simulink model "KV_Function_Valve"  (R2013b)
settings: Solver=ode45  StartTime=0.0  StopTime=10.0  RelTol=1e-3
libraries: simulink x1
settings Model: Creator=drhf  LastModifiedBy=drhf
settings OptimizationCC: InlineParams=on

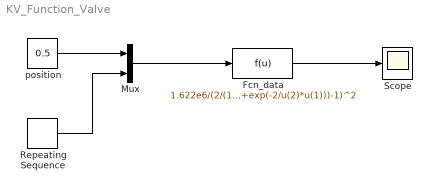
== system KV_Function_Valve ==
  Fcn_data : Fcn  Expr=1.622e6/(2/(1+exp(-2/u(2)*u(1)))-1)^2
  Mux : Mux  Inputs=2
  Repeating Sequence : simulink/Sources/Repeating Sequence  rep_seq_t=[0 10]  rep_seq_y=[0.5 10]
  Scope : Scope
  position : Constant  Value=0.5
  wires:
  Fcn_data/1 -> Scope/1
  position/1 -> Mux/1
  Mux/1 -> Fcn_data/1
  Repeating Sequence/1 -> Mux/2
